simulink subsystem "s_0303simulator"  (R2021a)
settings: Solver=VariableStepAuto  StartTime=0.0  StopTime=10.0  RelTol=1e-3
model mask{th_0=0, al_0=0, th_dot_0=0, al_dot_0=0}
  mask prompts: th_0 "Initial theta"; al_0 "Initial alpha"; th_dot_0 "Initial theta dot"; al_dot_0 "Initial alpha dot"
settings Model: Creator=paolo  LastModifiedBy=paolo

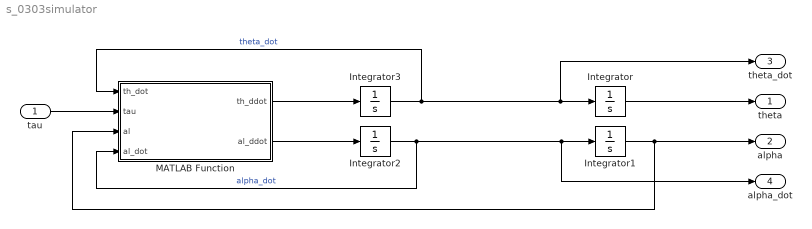
== system s_0303simulator ==
  tau : Inport
  Integrator : Integrator  InitialCondition=th_0  UpperSaturationLimit=pi/2  LowerSaturationLimit=-pi/2
  Integrator1 : Integrator  InitialCondition=al_0  UpperSaturationLimit=0.01  LowerSaturationLimit=-0.01
  Integrator2 : Integrator  InitialCondition=al_dot_0  UpperSaturationLimit=0.01  LowerSaturationLimit=-0.01
  Integrator3 : Integrator  InitialCondition=th_dot_0  UpperSaturationLimit=90  LowerSaturationLimit=-90
  MATLAB Function : MATLAB Function  TreatAsAtomicUnit=on
  theta : Outport
  alpha : Outport  Port=2
  theta_dot : Outport  Port=3
  alpha_dot : Outport  Port=4
  wires:
  Integrator/1 -> theta/1
  Integrator1/1 -> MATLAB Function/3(al), alpha/1
  Integrator2/1 -> MATLAB Function/4(al_dot), Integrator1/1, alpha_dot/1  "alpha_dot"
  Integrator3/1 -> Integrator/1, theta_dot/1, MATLAB Function/1(th_dot)  "theta_dot"
  MATLAB Function/1(th_ddot) -> Integrator3/1
  MATLAB Function/2(al_ddot) -> Integrator2/1
  tau/1 -> MATLAB Function/2(tau)

== matlab function s_0303simulator/MATLAB Function ==
  data: th_dot input; tau input; th_ddot output; al input; al_dot input; al_ddot output; PARAMS parameter
function [th_ddot, al_ddot] = dyn_model(th_dot, tau, al, al_dot, PARAMS)

    mp = PARAMS.mp;
    Lp = PARAMS.Lp;
    mr = PARAMS.mr;
    Lr = PARAMS.Lr;
    Jm = PARAMS.Jm;
    Jh = PARAMS.Jh;
    Cth = PARAMS.Cth;
    Cal = PARAMS.Cal;
    
    g = 9.81;
    
    a_11 = mp * (Lp^2/4 - Lp^2*cos(al)^2/4 + Lr^2) + mr*Lr^2/3 + Jm + Jh;
    a_12 = mp*Lp*Lr*cos(al)/2;
    a_21 = mp*Lp*Lr*cos(al)/2;
    a_22 = mp*Lp^2/3;
    
    det_A = (a_11*a_22 - a_12*a_21);
    
    b_1 = tau - Cth*th_dot - (mp*Lp^2*sin(2*al)/4)*al_dot*th_dot + ...
          (mp*Lp*Lr*sin(al)/2)*al_dot^2;
    b_2 = -Cal*al_dot - mp*g*Lp*sin(al)/2 + (mp*Lp^2*sin(2*al)/8)*th_dot^2;
    
    th_ddot = (b_1*a_22 - b_2*a_12) / det_A;
    al_ddot = (-b_1*a_21 + b_2*a_11) / det_A;
    
end
